simulink library "LDM_Controller"  (R2018b)
settings: Solver=VariableStepAuto  StartTime=0.0  StopTime=10.0  RelTol=1e-3
values from neighbouring files (symbols this model uses):
  K10_LDM_aOLCtrlerTableX : value not decoded    [LDM_DataDict.sldd]
  K10_LDM_torqOLCtrlerTableY : value not decoded    [LDM_DataDict.sldd]
  K_LDM_torqDecelClsCtrlerLowLim = -1000.0    [LDM_DataDict.sldd]
  K_LDM_torqDecelClsCtrlerUpLim = 1000.0    [LDM_DataDict.sldd]
  K_LDM_torqDecelCtrlerLowLim = 0.0    [LDM_DataDict.sldd]
  K_LDM_torqDecelCtrlerUpLim = 20000.0    [LDM_DataDict.sldd]
  K_LDM_torqOLCtrlerDecRate = 2.0    [LDM_DataDict.sldd]
  K_LDM_torqOLCtrlerIncRate = 2.0    [LDM_DataDict.sldd]
  K_LDM_torqOLCtrlerLowLim = 0.0    [LDM_DataDict.sldd]
  K_LDM_torqOLCtrlerResetLim = 10.0    [LDM_DataDict.sldd]
  K_LDM_torqOLCtrlerUpLim = 20000.0    [LDM_DataDict.sldd]
  LDM_VLD_EN_T : value not decoded    [LDM_DataDict.sldd]
  LDMCtrlMode_en_t : value not decoded    [LDM_DataDict.sldd]
undefined symbols (not defined in the file or in its folder): DiscIntNeverNeededParam
libraries: simulink x12
(part 2 of 2)

== stateflow chart LDM_Controller/Switch-Hybird Controller/LDM_Arbitrator ==
  state Decel_Control
    en:
    V_LDM_resetCtrler_bl = false;
    V_LDM_coHighSpdP = K_LDM_coDecelCtrlHighSpd_P;
    V_LDM_coHighSpdI = K_LDM_coDecelCtrlHighSpd_I;
    V_LDM_coLowSpdP = K_LDM_coDecelCtrlLowSpd_P;
    V_LDM_coLowSpdI = K_LDM_coDecelCtrlLowSpd_I;
    % PI parameters for DBR CST
    V_LDM_coCSTP = K_LDM_coDecelCtrlCST_P;
    V_LDM_coCSTI = K_LDM_coDecelCtrlCST_I;
    % PI parameters for EBR Self Brake
    V_LDM_coEbrSlfBrkP = K_LDM_coDecelCtrlEbrSB_P;
    V_LDM_coEbrSlfBrkI = K_LDM_coDecelCtrlEbrSB_I;
    state Standby
      % No brake request current VehAcc as the default value
      V_LDM_stBrkSrcMode_en = LDM_BRK_SRC_MODE_EN_T.BTA_PEDAL_BRAKE_NONE;
      V_LDM_aCtrlerSetpoint_f32 = single(0);
      V_LDM_coCtrlerPCoeff_f32 = single(0);
      V_LDM_coCtrlerICoeff_f32 = single(0);
      V_LDM_aCtrlErr_f32 = single(0);
      V_LDM_stBrkArbMode_en = LDMBrkArbMode_en_t.Standby;
      ex:
      V_LDM_resetCtrlerVal=single(V_LDM_PrvCtrlerOut);
    state EBR_control
      V_LDM_stBrkSrcMode_en = LDM_BRK_SRC_MODE_EN_T.BTA_EXTERNAL_BRAKE;
      V_LDM_aCtrlerSetpoint_f32 = V_EBR_aCHACCDecelReq;
      if V_LDM_stVehFwBw_en >= 0
      % moving forward or hold
      V_LDM_aVehAccDecLong = -V_VDS_aVehAccLong;
      else
      % moving backward
      V_LDM_aVehAccDecLong = V_VDS_aVehAccLong;
      end
      state EBR_Standby
        V_LDM_stBrkArbMode_en = LDMBrkArbMode_en_t.EBR_Standby;
        V_LDM_stCtrlMode_en = LDMCtrlMode_en_t.DecelCtrl;
        V_LDM_aCtrlerSetpoint_f32 = single(0);
        V_LDM_coCtrlerPCoeff_f32 = single(0);
        V_LDM_coCtrlerICoeff_f32 = single(0);
        V_LDM_aCtrlErr_f32 = single(0);
        V_LDM_resetCtrlerVal = single(0);
        V_LDM_resetCtrler_bl=~V_LDM_resetCtrler_bl;
      state EBR_DecelCtrl
        state DecelCtrl_CL_HighSpd
          en:
          V_LDM_stCtrlMode_en = LDMCtrlMode_en_t.DecelCtrl;
          V_LDM_coCtrlerPCoeff_f32 = V_LDM_coHighSpdP;
          V_LDM_coCtrlerICoeff_f32 = V_LDM_coHighSpdI;
          V_LDM_aCtrlErr_f32 = V_LDM_aCtrlerSetpoint_f32-V_LDM_aVehAccDecLong;
          V_LDM_resetCtrlerVal=V_LDM_PrvCtrlerOut-V_LDM_coCtrlerPCoeff_f32*V_LDM_aCtrlErr_f32;
          V_LDM_resetCtrler_bl=~V_LDM_resetCtrler_bl;
          du:
          V_LDM_aCtrlErr_f32 = V_LDM_aCtrlerSetpoint_f32-V_LDM_aVehAccDecLong;
        state DecelCtrl_CL_LowSpd
          en:
          V_LDM_stCtrlMode_en = LDMCtrlMode_en_t.DecelCtrl;
          V_LDM_coCtrlerPCoeff_f32 = V_LDM_coLowSpdP;
          V_LDM_coCtrlerICoeff_f32 = V_LDM_coLowSpdI;
          V_LDM_aCtrlErr_f32 = V_LDM_aCtrlerSetpoint_f32-V_LDM_aVehAccDecLong;
          V_LDM_resetCtrlerVal=V_LDM_PrvCtrlerOut-V_LDM_coCtrlerPCoeff_f32*V_LDM_aCtrlErr_f32;
          V_LDM_resetCtrler_bl=~V_LDM_resetCtrler_bl;
          du:
          V_LDM_aCtrlErr_f32 = V_LDM_aCtrlerSetpoint_f32-V_LDM_aVehAccDecLong;
        state DecelCtrl_OL
          en:
          V_LDM_stCtrlMode_en = LDMCtrlMode_en_t.OLCtrl; % open-loop control
          V_LDM_coCtrlerPCoeff_f32 = 0;
          V_LDM_coCtrlerICoeff_f32 = 0;
          V_LDM_resetCtrlerVal=V_LDM_PrvCtrlerOut;
          V_LDM_resetCtrler_bl=~V_LDM_resetCtrler_bl;
        (junction 414) -> Decel_Control.EBR_control.EBR_DecelCtrl.DecelCtrl_CL_HighSpd
        (junction 412) -> (junction 414) [order 2]
        Decel_Control.EBR_control.EBR_DecelCtrl.DecelCtrl_CL_HighSpd -> Decel_Control.EBR_control.EBR_DecelCtrl.DecelCtrl_CL_LowSpd : [abs(V_VDS_velVehSpd) <= K_LDM_coDecelCtrlHigh2LowLim]
        Decel_Control.EBR_control.EBR_DecelCtrl.DecelCtrl_CL_LowSpd -> Decel_Control.EBR_control.EBR_DecelCtrl.DecelCtrl_CL_HighSpd [order 2] : [abs(V_VDS_velVehSpd) > K_LDM_coDecelCtrlLow2HighLim]
        (junction 412) -> Decel_Control.EBR_control.EBR_DecelCtrl.DecelCtrl_CL_LowSpd [order 1] : [abs(V_VDS_velVehSpd) <= K_LDM_coDecelCtrlHigh2LowLim]
        (junction 411) -> (junction 412) [order 2]
        Decel_Control.EBR_control.EBR_DecelCtrl.DecelCtrl_OL -> Decel_Control.EBR_control.EBR_DecelCtrl.DecelCtrl_CL_LowSpd : [abs(V_VDS_velVehSpd) > K_LDM_coDecelCtrlOl2ClLim && ...
            | K_LDM_blClsLoopCtrlEnable_bl == true]
        Decel_Control.EBR_control.EBR_DecelCtrl.DecelCtrl_CL_LowSpd -> Decel_Control.EBR_control.EBR_DecelCtrl.DecelCtrl_OL [order 1] : [abs(V_VDS_velVehSpd) <= K_LDM_coDecelCtrlCl2OlLim]
        (junction 411) -> Decel_Control.EBR_control.EBR_DecelCtrl.DecelCtrl_OL [order 1] : [abs(V_VDS_velVehSpd) <= K_LDM_coDecelCtrlCl2OlLim || ...
            | K_LDM_blClsLoopCtrlEnable_bl == false]
        (default) -> (junction 411)
      state SelfBrake
        V_LDM_aCtrlErr_f32 = V_LDM_aCtrlerSetpoint_f32-V_LDM_aVehAccDecLong;
        state SelfBrake_follow
          en:
          V_LDM_stCtrlMode_en = LDMCtrlMode_en_t.DecelCtrl;
          V_LDM_coCtrlerPCoeff_f32 = V_LDM_coEbrSlfBrkP;
          V_LDM_coCtrlerICoeff_f32 = V_LDM_coEbrSlfBrkI;
          V_LDM_resetCtrlerVal=V_LDM_PrvCtrlerOut-V_LDM_coCtrlerPCoeff_f32*V_LDM_aCtrlErr_f32;
          V_LDM_resetCtrler_bl=~V_LDM_resetCtrler_bl;
        state StableJudge
          en:
          V_LDM_stCtrlMode_en = LDMCtrlMode_en_t.OLCtrl; % open-loop control
          V_LDM_coCtrlerPCoeff_f32 = 0;
          V_LDM_coCtrlerICoeff_f32 = 0;
          V_LDM_resetCtrlerVal=V_LDM_PrvCtrlerOut;
          V_LDM_resetCtrler_bl=~V_LDM_resetCtrler_bl;
        (junction 426) -> SelfBrake_follow
        (junction 424) -> (junction 426) [order 2]
        SelfBrake_follow -> StableJudge : [abs(V_VDS_velVehSpd) <= K_LDM_coDecelCtrlCl2OlLim]
        StableJudge -> SelfBrake_follow : [abs(V_VDS_velVehSpd) > K_LDM_coDecelCtrlOl2ClLim && ...
            | K_LDM_blClsLoopCtrlEnable_bl == true]
        (junction 424) -> StableJudge [order 1] : [abs(V_VDS_velVehSpd) <= K_LDM_coDecelCtrlCl2OlLim || ...
            | K_LDM_blClsLoopCtrlEnable_bl == false]
        (default) -> (junction 424)
      state HoldPressure
        en:
        V_LDM_stCtrlMode_en = LDMCtrlMode_en_t.OLCtrl;
        V_LDM_coCtrlerPCoeff_f32 = 0;
        V_LDM_coCtrlerICoeff_f32 = 0;
        V_LDM_resetCtrlerVal=V_LDM_PrvCtrlerOut;
        V_LDM_resetCtrler_bl=~V_LDM_resetCtrler_bl;
      (default) -> (junction 128)
      (junction 128) -> EBR_Standby [order 1] : [V_EBR_stCHACCRunbleSts_en == CHACCRunbleSts_en_t.ACC_standby]
      EBR_Standby -> EBR_control : [V_EBR_stCHACCRunbleSts_en ~= CHACCRunbleSts_en_t.ACC_standby]
      (junction 128) -> (junction 150) [order 2]
      (junction 225) -> EBR_Standby
      (junction 226) -> (junction 225) : {V_LDM_stBrkArbMode_en = LDMBrkArbMode_en_t.EBR_Error;}%error
      (junction 150) -> EBR_DecelCtrl [order 1] : [V_EBR_stCHACCRunbleSts_en == CHACCRunbleSts_en_t.ACC_CB]
          | {V_LDM_stBrkArbMode_en = LDMBrkArbMode_en_t.EBR_NormCtrl;}
      (junction 150) -> (junction 291) [order 2]
      EBR_DecelCtrl -> EBR_control : [V_EBR_stCHACCRunbleSts_en ~= CHACCRunbleSts_en_t.ACC_CB]
      (junction 291) -> SelfBrake [order 1] : [V_EBR_stCHACCRunbleSts_en == CHACCRunbleSts_en_t.ACC_SB]
          | {V_LDM_stBrkArbMode_en = LDMBrkArbMode_en_t.EBR_SelfBrake;}
      (junction 291) -> (junction 149) [order 2]
      SelfBrake -> EBR_control : [V_EBR_stCHACCRunbleSts_en ~= CHACCRunbleSts_en_t.ACC_SB]
      Decel_Control.EBR_control.HoldPressure -> EBR_control : [V_EBR_stCHACCRunbleSts_en ~= CHACCRunbleSts_en_t.ACC_HOLD]
      (junction 149) -> Decel_Control.EBR_control.HoldPressure [order 1] : [V_EBR_stCHACCRunbleSts_en == CHACCRunbleSts_en_t.ACC_HOLD]
      (junction 149) -> (junction 226) [order 2]
    state DBR_control
      V_LDM_stBrkSrcMode_en = LDM_BRK_SRC_MODE_EN_T.BTA_PEDAL_APPLIED;
      V_LDM_aCtrlerSetpoint_f32 = V_DBR_aDBRDecelReq;
      if V_LDM_stVehFwBw_en >= 0
      % moving forward or hold
      V_LDM_aVehAccDecLong = -V_VDS_aVehAccLong;
      else
      % moving backward
      V_LDM_aVehAccDecLong = V_VDS_aVehAccLong;
      end
      state initial
        V_LDM_stBrkArbMode_en = LDMBrkArbMode_en_t.DBR_Init;
      state DBR_DecelCtrl
        state DecelCtrl_CL_HighSpd
          en:
          V_LDM_stCtrlMode_en = LDMCtrlMode_en_t.DecelCtrl;
          V_LDM_coCtrlerPCoeff_f32 = V_LDM_coHighSpdP;
          V_LDM_coCtrlerICoeff_f32 = V_LDM_coHighSpdI;
          V_LDM_aCtrlErr_f32 = V_LDM_aCtrlerSetpoint_f32-V_LDM_aVehAccDecLong;
          V_LDM_resetCtrlerVal=V_LDM_PrvCtrlerOut-V_LDM_coCtrlerPCoeff_f32*V_LDM_aCtrlErr_f32;
          V_LDM_resetCtrler_bl=~V_LDM_resetCtrler_bl;
          du:
          V_LDM_aCtrlErr_f32 = V_LDM_aCtrlerSetpoint_f32-V_LDM_aVehAccDecLong;
        state DecelCtrl_CL_LowSpd
          en:
          V_LDM_stCtrlMode_en = LDMCtrlMode_en_t.DecelCtrl;
          V_LDM_coCtrlerPCoeff_f32 = V_LDM_coLowSpdP;
          V_LDM_coCtrlerICoeff_f32 = V_LDM_coLowSpdI;
          V_LDM_aCtrlErr_f32 = V_LDM_aCtrlerSetpoint_f32-V_LDM_aVehAccDecLong;
          V_LDM_resetCtrlerVal=V_LDM_PrvCtrlerOut-V_LDM_coCtrlerPCoeff_f32*V_LDM_aCtrlErr_f32;
          V_LDM_resetCtrler_bl=~V_LDM_resetCtrler_bl;
          du:
          V_LDM_aCtrlErr_f32 = V_LDM_aCtrlerSetpoint_f32-V_LDM_aVehAccDecLong;
        state DecelCtrl_OL
          en:
          V_LDM_stCtrlMode_en = LDMCtrlMode_en_t.OLCtrl; % open-loop control
          V_LDM_coCtrlerPCoeff_f32 = 0;
          V_LDM_coCtrlerICoeff_f32 = 0;
          V_LDM_resetCtrlerVal=V_LDM_PrvCtrlerOut;
          V_LDM_resetCtrler_bl=~V_LDM_resetCtrler_bl;
        (junction 389) -> Decel_Control.DBR_control.DBR_DecelCtrl.DecelCtrl_CL_HighSpd
        (junction 391) -> (junction 389) [order 2]
        Decel_Control.DBR_control.DBR_DecelCtrl.DecelCtrl_CL_HighSpd -> Decel_Control.DBR_control.DBR_DecelCtrl.DecelCtrl_CL_LowSpd : [abs(V_VDS_velVehSpd) <= K_LDM_coDecelCtrlHigh2LowLim]
        Decel_Control.DBR_control.DBR_DecelCtrl.DecelCtrl_CL_LowSpd -> Decel_Control.DBR_control.DBR_DecelCtrl.DecelCtrl_CL_HighSpd [order 2] : [abs(V_VDS_velVehSpd) > K_LDM_coDecelCtrlLow2HighLim]
        (junction 391) -> Decel_Control.DBR_control.DBR_DecelCtrl.DecelCtrl_CL_LowSpd [order 1] : [abs(V_VDS_velVehSpd) <= K_LDM_coDecelCtrlHigh2LowLim]
        (junction 393) -> (junction 391) [order 2]
        Decel_Control.DBR_control.DBR_DecelCtrl.DecelCtrl_OL -> Decel_Control.DBR_control.DBR_DecelCtrl.DecelCtrl_CL_LowSpd : [abs(V_VDS_velVehSpd) > K_LDM_coDecelCtrlOl2ClLim && ...
            | K_LDM_blClsLoopCtrlEnable_bl == true]
        Decel_Control.DBR_control.DBR_DecelCtrl.DecelCtrl_CL_LowSpd -> Decel_Control.DBR_control.DBR_DecelCtrl.DecelCtrl_OL [order 1] : [abs(V_VDS_velVehSpd) <= K_LDM_coDecelCtrlCl2OlLim]
        (junction 393) -> Decel_Control.DBR_control.DBR_DecelCtrl.DecelCtrl_OL [order 1] : [abs(V_VDS_velVehSpd) <= K_LDM_coDecelCtrlCl2OlLim || ...
            | K_LDM_blClsLoopCtrlEnable_bl == false]
        (default) -> (junction 393)
      state DBR_CST
        V_LDM_aCtrlErr_f32 = V_LDM_aCtrlerSetpoint_f32-V_LDM_aVehAccDecLong;
        state CST_follow
          en:
          V_LDM_stCtrlMode_en = LDMCtrlMode_en_t.DecelCtrl;
          V_LDM_coCtrlerPCoeff_f32 = V_LDM_coCSTP;
          V_LDM_coCtrlerICoeff_f32 = V_LDM_coCSTI;
          V_LDM_resetCtrlerVal=V_LDM_PrvCtrlerOut-V_LDM_coCtrlerPCoeff_f32*V_LDM_aCtrlErr_f32;
          V_LDM_resetCtrler_bl=~V_LDM_resetCtrler_bl;
        state CST_OL
          en:
          V_LDM_stCtrlMode_en = LDMCtrlMode_en_t.OLCtrl; % open-loop control
          V_LDM_coCtrlerPCoeff_f32 = 0;
          V_LDM_coCtrlerICoeff_f32 = 0;
          V_LDM_resetCtrlerVal=V_LDM_PrvCtrlerOut;
          V_LDM_resetCtrler_bl=~V_LDM_resetCtrler_bl;
        (junction 421) -> CST_follow
        (junction 419) -> (junction 421) [order 2]
        CST_follow -> CST_OL : [abs(V_VDS_velVehSpd) <= K_LDM_coDecelCtrlCl2OlLim]
        CST_OL -> CST_follow : [abs(V_VDS_velVehSpd) >= K_LDM_coDecelCtrlOl2ClLim && ...
            | K_LDM_blClsLoopCtrlEnable_bl == true]
        (junction 419) -> CST_OL [order 1] : [abs(V_VDS_velVehSpd) <= K_LDM_coDecelCtrlCl2OlLim || ...
            | K_LDM_blClsLoopCtrlEnable_bl == false]
        (default) -> (junction 419)
      state HoldPressure
        en:
        V_LDM_stBrkArbMode_en = LDMBrkArbMode_en_t.DBR_HldPres;
        V_LDM_stCtrlMode_en = LDMCtrlMode_en_t.OLCtrl;
        V_LDM_coCtrlerPCoeff_f32 = 0;
        V_LDM_coCtrlerICoeff_f32 = 0;
        V_LDM_resetCtrlerVal=V_LDM_PrvCtrlerOut;
        V_LDM_resetCtrler_bl=~V_LDM_resetCtrler_bl;
      (default) -> (junction 211)
      initial -> DBR_control : [V_DBR_stDBRRunbleSts_en ~= DBRCSTRunbleSts_en_t.initial]
      (junction 211) -> initial [order 1] : [V_DBR_stDBRRunbleSts_en == DBRCSTRunbleSts_en_t.initial]
      (junction 211) -> (junction 181) [order 2]
      (junction 181) -> DBR_DecelCtrl [order 1] : [V_DBR_stDBRRunbleSts_en == DBRCSTRunbleSts_en_t.CST_emergency_control]
          | {V_LDM_stBrkArbMode_en = LDMBrkArbMode_en_t.DBR_EmergCtrl;}
      (junction 181) -> (junction 180) [order 2]
      DBR_DecelCtrl -> DBR_control : [V_DBR_stDBRRunbleSts_en ~= DBRCSTRunbleSts_en_t.dynamic_control &&...
          | V_DBR_stDBRRunbleSts_en ~= DBRCSTRunbleSts_en_t.CST_standby_dynamic_control &&...
          | V_DBR_stDBRRunbleSts_en ~= DBRCSTRunbleSts_en_t.CST_emergency_control]
      (junction 180) -> DBR_DecelCtrl [order 1] : [V_DBR_stDBRRunbleSts_en == DBRCSTRunbleSts_en_t.dynamic_control ||...
          | V_DBR_stDBRRunbleSts_en == DBRCSTRunbleSts_en_t.CST_standby_dynamic_control]
          | {V_LDM_stBrkArbMode_en = LDMBrkArbMode_en_t.DBR_NormCtrl;}
      (junction 180) -> (junction 182) [order 2]
      (junction 262) -> DBR_DecelCtrl
      (junction 260) -> (junction 262) : {V_LDM_stBrkArbMode_en = LDMBrkArbMode_en_t.DBR_Error;}%error
      DBR_CST -> DBR_control : [V_DBR_stDBRRunbleSts_en ~= DBRCSTRunbleSts_en_t.CST_active]
      (junction 182) -> DBR_CST [order 1] : [V_DBR_stDBRRunbleSts_en == DBRCSTRunbleSts_en_t.CST_active]
          | {V_LDM_stBrkArbMode_en = LDMBrkArbMode_en_t.DBR_CST;}
      (junction 182) -> (junction 273) [order 2]
      Decel_Control.DBR_control.HoldPressure -> DBR_control : [V_DBR_stDBRRunbleSts_en ~= DBRCSTRunbleSts_en_t.CST_off && ...
          | V_DBR_stDBRRunbleSts_en ~= DBRCSTRunbleSts_en_t.CST_standby_standstill_control &&...
          | V_DBR_stDBRRunbleSts_en ~= DBRCSTRunbleSts_en_t.standstill_control]
      (junction 273) -> Decel_Control.DBR_control.HoldPressure [order 1] : [V_DBR_stDBRRunbleSts_en == DBRCSTRunbleSts_en_t.CST_off ||...
          | V_DBR_stDBRRunbleSts_en == DBRCSTRunbleSts_en_t.CST_standby_standstill_control ||...
          | V_DBR_stDBRRunbleSts_en == DBRCSTRunbleSts_en_t.standstill_control]
      (junction 273) -> (junction 260) [order 2]
    DBR_control -> Standby [order 1] : [V_DBR_EBR_stBrkArbMode_en==BrkArbMode_en_t.brake_no_request]
        | {V_LDM_resetCtrler_bl=~V_LDM_resetCtrler_bl; V_LDM_resetCtrlerVal=single(0);}
    EBR_control -> Standby [order 1] : [V_DBR_EBR_stBrkArbMode_en==BrkArbMode_en_t.brake_no_request]
        | {V_LDM_resetCtrler_bl=~V_LDM_resetCtrler_bl; V_LDM_resetCtrlerVal=single(0);}
    Standby -> DBR_control [order 1] : [V_DBR_EBR_stBrkArbMode_en==BrkArbMode_en_t.DBR_arbitration]
    Standby -> EBR_control [order 2] : [V_DBR_EBR_stBrkArbMode_en==BrkArbMode_en_t.ACC_arbitration && ...
        | V_EBR_stCHACCRunbleSts_en ~= CHACCRunbleSts_en_t.ACC_off]
    (junction 71) -> Standby [order 3]
    (junction 71) -> EBR_control [order 2] : [V_DBR_EBR_stBrkArbMode_en==BrkArbMode_en_t.ACC_arbitration]
    (junction 71) -> DBR_control [order 1] : [V_DBR_EBR_stBrkArbMode_en==BrkArbMode_en_t.DBR_arbitration]
    (default) -> (junction 71)
    DBR_control -> EBR_control [order 2] : [V_DBR_EBR_stBrkArbMode_en==BrkArbMode_en_t.ACC_arbitration]
    EBR_control -> DBR_control [order 2] : [V_DBR_EBR_stBrkArbMode_en==BrkArbMode_en_t.DBR_arbitration]
  (default) -> Decel_Control
  data: V_LDM_stCtrlMode_en output; V_LDM_aCtrlErr_f32 output; V_DBR_EBR_stBrkArbMode_en input Enum: BrkArbMode_en_t; V_LDM_stVehFwBw_en input Enum: LDMVehFwBw_en_t; V_DBR_aDBRDecelReq input single; V_EBR_aCHACCDecelReq input single; V_DBR_stDBRRunbleSts_en input Enum: DBRCSTRunbleSts_en_t; V_EBR_stCHACCRunbleSts_en input Enum: CHACCRunbleSts_en_t; V_VDS_aVehAccLong input single; V_VDS_velVehSpd input single; V_LDM_coCtrlerPCoeff_f32 output single; V_LDM_coCtrlerICoeff_f32 output single; V_LDM_resetCtrler_bl output boolean; V_LDM_resetCtrlerVal output single; V_LDM_PrvCtrlerOut input single; V_LDM_aCtrlerSetpoint_f32 output single; V_LDM_coHighSpdI local single; V_LDM_coHighSpdP local single; V_LDM_coCSTI local single; V_LDM_aVehAccDecLong local single; V_LDM_coCSTP local; V_LDM_stBrkArbMode_en output; K_LDM_coDecelCtrlCST_I parameter; K_LDM_coDecelCtrlCST_P parameter; V_LDM_coEbrSlfBrkP local; V_LDM_coEbrSlfBrkI local; K_LDM_coDecelCtrlEbrSB_I parameter; K_LDM_coDecelCtrlEbrSB_P parameter; V_LDM_coLowSpdI local; V_LDM_coLowSpdP local; K_LDM_coDecelCtrlHighSpd_I parameter; K_LDM_coDecelCtrlLowSpd_I parameter; K_LDM_coDecelCtrlHighSpd_P parameter; K_LDM_coDecelCtrlLowSpd_P parameter; K_LDM_coDecelCtrlCl2OlLim parameter; K_LDM_coDecelCtrlHigh2LowLim parameter; K_LDM_coDecelCtrlLow2HighLim parameter; K_LDM_coDecelCtrlOl2ClLim parameter; K_LDM_blClsLoopCtrlEnable_bl parameter; V_LDM_stBrkSrcMode_en output

== stateflow chart LDM_Controller/Switch-Hybird Controller/Decel open-loop controler1/reset ==
  state CalDiff
    en:
    if PrevCtrlOutput <= 0.1 || K_LDM_blClsLoopCtrlEnable_bl == false
    %previous control output equals zero, or closed loop control is unabled
    eta = 1;
    else
    eta = PrevCtrlOutput / max(1, LookupTableValue);
    end
  state Hold
  (default) -> CalDiff
  CalDiff -> Hold : [~enable]
  Hold -> CalDiff : [enable]
  data: enable input boolean; LookupTableValue input single; PrevCtrlOutput input single; eta output single; K_LDM_blClsLoopCtrlEnable_bl parameter

== stateflow chart LDM_Controller/Parallel-Hybird Controller/Decel open-loop controler1/reset ==
  state CalDiff
    en:
    if PrevCtrlOutput <= 0.1 || K_LDM_blClsLoopCtrlEnable_bl == false
    %previous control output equals zero, or closed loop control is unabled
    eta = 1;
    else
    eta = PrevCtrlOutput / max(1, LookupTableValue);
    end
  state Hold
  (default) -> CalDiff
  CalDiff -> Hold : [~enable]
  Hold -> CalDiff : [enable]
  data: enable input boolean; LookupTableValue input single; PrevCtrlOutput input single; eta output single; K_LDM_blClsLoopCtrlEnable_bl parameter

== stateflow chart LDM_Controller/Parallel-Hybird Controller/LDM_Arbitrator ==
  state Decel_Control
    en:
    V_LDM_resetCtrler_bl = false;
    V_LDM_coHighSpdP = K_LDM_coDecelParalCtrlHighSpd_P;
    V_LDM_coHighSpdI = K_LDM_coDecelParalCtrlHighSpd_I;
    V_LDM_coLowSpdP = K_LDM_coDecelParalCtrlLowSpd_P;
    V_LDM_coLowSpdI = K_LDM_coDecelParalCtrlLowSpd_I;
    % PI parameters for DBR CST
    V_LDM_coCSTP = K_LDM_coDecelParalCtrlCST_P;
    V_LDM_coCSTI = K_LDM_coDecelParalCtrlCST_I;
    % PI parameters for EBR Self Brake
    V_LDM_coEbrSlfBrkP = K_LDM_coDecelParalCtrlEbrSB_P;
    V_LDM_coEbrSlfBrkI = K_LDM_coDecelParalCtrlEbrSB_I;
    du:
    % whether enable the closed loop controller
    if K_LDM_blClsLoopCtrlEnable_bl == false
    V_LDM_stClsLoopEnable = false;
    else
    if V_LDM_stVehFwBw_en == LDMVehFwBw_en_t.Forward ||...
    V_LDM_stVehFwBw_en == LDMVehFwBw_en_t.Backward
    V_LDM_stClsLoopEnable = true;
    else
    V_LDM_stClsLoopEnable = false;
    end
    end
    % moving forward
    if V_LDM_stVehFwBw_en == LDMVehFwBw_en_t.Forward
    V_LDM_aVehAccDecLong = -V_VDS_aVehAccLong;
    % moving backward
    elseif V_LDM_stVehFwBw_en == LDMVehFwBw_en_t.Backward
    V_LDM_aVehAccDecLong = V_VDS_aVehAccLong;
    else
    V_LDM_aVehAccDecLong = V_VDS_aVehAccLong;
    end
    V_LDM_aVehAccErr = V_LDM_aCtrlerSetpoint_f32-V_LDM_aVehAccDecLong;
    state Standby
      % No brake request current VehAcc as the default value
      V_LDM_stBrkSrcMode_en = LDM_BRK_SRC_MODE_EN_T.BTA_PEDAL_BRAKE_NONE;
      V_LDM_aCtrlerSetpoint_f32 = single(0);
      V_LDM_coCtrlerPCoeff_f32 = single(0);
      V_LDM_coCtrlerICoeff_f32 = single(0);
      V_LDM_aCtrlErr_f32 = single(0);
      V_LDM_stBrkArbMode_en = LDMBrkArbMode_en_t.Standby;
      en:
      V_LDM_resetCtrlerVal = single(0);
      V_LDM_resetCtrler_bl=~V_LDM_resetCtrler_bl;
      ex:
      V_LDM_resetCtrlerVal=single(V_LDM_PrvClsLoopCtrlerOut);
    state DBR_control
      V_LDM_stBrkSrcMode_en = LDM_BRK_SRC_MODE_EN_T.BTA_PEDAL_APPLIED;
      V_LDM_aCtrlerSetpoint_f32 = V_DBR_aDBRDecelReq;
      state initial
        V_LDM_stBrkArbMode_en = LDMBrkArbMode_en_t.DBR_Init;
        V_LDM_stCtrlMode_en = LDMCtrlMode_en_t.OLCtrl;
      state DBR_DecelCtrl
        state DecelCtrl_CL_HighSpd
          en,du:
          V_LDM_aCtrlErr_f32 = V_LDM_aVehAccErr;
          en:
          V_LDM_stCtrlMode_en = LDMCtrlMode_en_t.DecelCtrl;
          V_LDM_coCtrlerPCoeff_f32 = V_LDM_coHighSpdP;
          V_LDM_coCtrlerICoeff_f32 = V_LDM_coHighSpdI;
          V_LDM_resetCtrlerVal=V_LDM_PrvClsLoopCtrlerOut-V_LDM_coCtrlerPCoeff_f32*V_LDM_aCtrlErr_f32;
          V_LDM_resetCtrler_bl=~V_LDM_resetCtrler_bl;
        state DecelCtrl_CL_LowSpd
          en,du:
          V_LDM_aCtrlErr_f32 = V_LDM_aVehAccErr;
          en:
          V_LDM_stCtrlMode_en = LDMCtrlMode_en_t.DecelCtrl;
          V_LDM_coCtrlerPCoeff_f32 = V_LDM_coLowSpdP;
          V_LDM_coCtrlerICoeff_f32 = V_LDM_coLowSpdI;
          V_LDM_resetCtrlerVal=V_LDM_PrvClsLoopCtrlerOut-V_LDM_coCtrlerPCoeff_f32*V_LDM_aCtrlErr_f32;
          V_LDM_resetCtrler_bl=~V_LDM_resetCtrler_bl;
        state DecelCtrl_OL
          en:
          V_LDM_coCtrlerPCoeff_f32 = 0;
          V_LDM_coCtrlerICoeff_f32 = V_LDM_coLowSpdI / V_LDM_coLowSpdP;
          V_LDM_resetCtrlerVal=V_LDM_PrvClsLoopCtrlerOut;
          V_LDM_resetCtrler_bl=~V_LDM_resetCtrler_bl;
          du:
          V_LDM_aCtrlErr_f32 = - V_LDM_PrvClsLoopCtrlerOut; % let cls ctrl go to zero smoothly
          if abs(V_LDM_PrvClsLoopCtrlerOut) <= 0.1
          V_LDM_stCtrlMode_en = LDMCtrlMode_en_t.OLCtrl; % open-loop control
          V_LDM_coCtrlerICoeff_f32 = 0;
          V_LDM_resetCtrlerVal=0;
          V_LDM_resetCtrler_bl=~V_LDM_resetCtrler_bl;
          end
        (junction 389) -> Decel_Control.DBR_control.DBR_DecelCtrl.DecelCtrl_CL_HighSpd
        (junction 391) -> (junction 389) [order 2]
        Decel_Control.DBR_control.DBR_DecelCtrl.DecelCtrl_CL_HighSpd -> Decel_Control.DBR_control.DBR_DecelCtrl.DecelCtrl_CL_LowSpd : [abs(V_VDS_velVehSpd) <= K_LDM_coDecelCtrlHigh2LowLim]
        Decel_Control.DBR_control.DBR_DecelCtrl.DecelCtrl_CL_LowSpd -> Decel_Control.DBR_control.DBR_DecelCtrl.DecelCtrl_CL_HighSpd [order 2] : [abs(V_VDS_velVehSpd) > K_LDM_coDecelCtrlLow2HighLim]
        (junction 391) -> Decel_Control.DBR_control.DBR_DecelCtrl.DecelCtrl_CL_LowSpd [order 1] : [abs(V_VDS_velVehSpd) <= K_LDM_coDecelCtrlHigh2LowLim]
        (junction 393) -> (junction 391) [order 2]
        Decel_Control.DBR_control.DBR_DecelCtrl.DecelCtrl_OL -> Decel_Control.DBR_control.DBR_DecelCtrl.DecelCtrl_CL_LowSpd : [abs(V_VDS_velVehSpd) > K_LDM_coDecelCtrlOl2ClLim && ...
            | V_LDM_stClsLoopEnable == true]
        Decel_Control.DBR_control.DBR_DecelCtrl.DecelCtrl_CL_LowSpd -> Decel_Control.DBR_control.DBR_DecelCtrl.DecelCtrl_OL [order 1] : [abs(V_VDS_velVehSpd) <= K_LDM_coDecelCtrlCl2OlLim]
        (junction 393) -> Decel_Control.DBR_control.DBR_DecelCtrl.DecelCtrl_OL [order 1] : [abs(V_VDS_velVehSpd) <= K_LDM_coDecelCtrlCl2OlLim || ...
            | V_LDM_stClsLoopEnable == false]
        (default) -> (junction 393)
      state DBR_CST
        state CST_follow
          en,du:
          V_LDM_aCtrlErr_f32 = V_LDM_aVehAccErr;
          en:
          V_LDM_stCtrlMode_en = LDMCtrlMode_en_t.DecelCtrl;
          V_LDM_coCtrlerPCoeff_f32 = V_LDM_coCSTP;
          V_LDM_coCtrlerICoeff_f32 = V_LDM_coCSTI;
          V_LDM_resetCtrlerVal=V_LDM_PrvClsLoopCtrlerOut-V_LDM_coCtrlerPCoeff_f32*V_LDM_aCtrlErr_f32;
          V_LDM_resetCtrler_bl=~V_LDM_resetCtrler_bl;
        state CST_OL
          en:
          V_LDM_resetCtrlerVal=V_LDM_PrvClsLoopCtrlerOut;
          V_LDM_resetCtrler_bl=~V_LDM_resetCtrler_bl;
          V_LDM_coCtrlerPCoeff_f32 = 0;
          V_LDM_coCtrlerICoeff_f32 = V_LDM_coCSTI / V_LDM_coCSTP;
          du:
          V_LDM_aCtrlErr_f32 = - V_LDM_PrvClsLoopCtrlerOut; % let cls ctrl go to zero smoothly
          if abs(V_LDM_PrvClsLoopCtrlerOut) <= 0.1
          V_LDM_stCtrlMode_en = LDMCtrlMode_en_t.OLCtrl; % open-loop control
          V_LDM_coCtrlerICoeff_f32 = 0;
          V_LDM_resetCtrlerVal=0;
          V_LDM_resetCtrler_bl=~V_LDM_resetCtrler_bl;
          end
        (junction 421) -> CST_follow
        (junction 419) -> (junction 421) [order 2]
        CST_follow -> CST_OL : [abs(V_VDS_velVehSpd) <= K_LDM_coDecelCtrlCl2OlLim]
        CST_OL -> CST_follow : [abs(V_VDS_velVehSpd) >= K_LDM_coDecelCtrlOl2ClLim && ...
            | V_LDM_stClsLoopEnable == true]
        (junction 419) -> CST_OL [order 1] : [abs(V_VDS_velVehSpd) <= K_LDM_coDecelCtrlCl2OlLim || ...
            | V_LDM_stClsLoopEnable == false]
        (default) -> (junction 419)
      state HoldPressure
        en:
        V_LDM_stBrkArbMode_en = LDMBrkArbMode_en_t.DBR_HldPres;
        V_LDM_stCtrlMode_en = LDMCtrlMode_en_t.OLCtrl;
        V_LDM_coCtrlerPCoeff_f32 = 0;
        V_LDM_coCtrlerICoeff_f32 = 0;
        V_LDM_resetCtrlerVal=0;
        V_LDM_resetCtrler_bl=~V_LDM_resetCtrler_bl;
      (default) -> (junction 211)
      initial -> DBR_control : [V_DBR_stDBRRunbleSts_en ~= DBRCSTRunbleSts_en_t.initial]
      (junction 211) -> initial [order 1] : [V_DBR_stDBRRunbleSts_en == DBRCSTRunbleSts_en_t.initial]
      (junction 211) -> (junction 181) [order 2]
      (junction 181) -> DBR_DecelCtrl [order 1] : [V_DBR_stDBRRunbleSts_en == DBRCSTRunbleSts_en_t.CST_emergency_control]
          | {V_LDM_stBrkArbMode_en = LDMBrkArbMode_en_t.DBR_EmergCtrl;}
      (junction 181) -> (junction 180) [order 2]
      DBR_DecelCtrl -> DBR_control : [V_DBR_stDBRRunbleSts_en ~= DBRCSTRunbleSts_en_t.dynamic_control &&...
          | V_DBR_stDBRRunbleSts_en ~= DBRCSTRunbleSts_en_t.CST_standby_dynamic_control &&...
          | V_DBR_stDBRRunbleSts_en ~= DBRCSTRunbleSts_en_t.CST_emergency_control]
      (junction 180) -> DBR_DecelCtrl [order 1] : [V_DBR_stDBRRunbleSts_en == DBRCSTRunbleSts_en_t.dynamic_control ||...
          | V_DBR_stDBRRunbleSts_en == DBRCSTRunbleSts_en_t.CST_standby_dynamic_control]
          | {V_LDM_stBrkArbMode_en = LDMBrkArbMode_en_t.DBR_NormCtrl;}
      (junction 180) -> (junction 182) [order 2]
      (junction 262) -> DBR_DecelCtrl
      (junction 260) -> (junction 262) : {V_LDM_stBrkArbMode_en = LDMBrkArbMode_en_t.DBR_Error;}%error
      DBR_CST -> DBR_control : [V_DBR_stDBRRunbleSts_en ~= DBRCSTRunbleSts_en_t.CST_active]
      (junction 182) -> DBR_CST [order 1] : [V_DBR_stDBRRunbleSts_en == DBRCSTRunbleSts_en_t.CST_active]
          | {V_LDM_stBrkArbMode_en = LDMBrkArbMode_en_t.DBR_CST;}
      (junction 182) -> (junction 273) [order 2]
      Decel_Control.DBR_control.HoldPressure -> DBR_control : [V_DBR_stDBRRunbleSts_en ~= DBRCSTRunbleSts_en_t.CST_off && ...
          | V_DBR_stDBRRunbleSts_en ~= DBRCSTRunbleSts_en_t.CST_standby_standstill_control &&...
          | V_DBR_stDBRRunbleSts_en ~= DBRCSTRunbleSts_en_t.standstill_control]
      (junction 273) -> Decel_Control.DBR_control.HoldPressure [order 1] : [V_DBR_stDBRRunbleSts_en == DBRCSTRunbleSts_en_t.CST_off ||...
          | V_DBR_stDBRRunbleSts_en == DBRCSTRunbleSts_en_t.CST_standby_standstill_control ||...
          | V_DBR_stDBRRunbleSts_en == DBRCSTRunbleSts_en_t.standstill_control]
      (junction 273) -> (junction 260) [order 2]
    state EBR_control
      V_LDM_stBrkSrcMode_en = LDM_BRK_SRC_MODE_EN_T.BTA_EXTERNAL_BRAKE;
      V_LDM_aCtrlerSetpoint_f32 = V_EBR_aCHACCDecelReq;
      state EBR_Standby
        V_LDM_stBrkArbMode_en = LDMBrkArbMode_en_t.EBR_Standby;
        V_LDM_stCtrlMode_en = LDMCtrlMode_en_t.OLCtrl;
        V_LDM_aCtrlerSetpoint_f32 = single(0);
        V_LDM_coCtrlerPCoeff_f32 = single(0);
        V_LDM_coCtrlerICoeff_f32 = single(0);
        V_LDM_aCtrlErr_f32 = single(0);
        V_LDM_resetCtrlerVal = single(0);
        V_LDM_resetCtrler_bl=~V_LDM_resetCtrler_bl;
      state EBR_DecelCtrl
        state DecelCtrl_CL_HighSpd
          V_LDM_aCtrlErr_f32 = V_LDM_aVehAccErr;
          en:
          V_LDM_stCtrlMode_en = LDMCtrlMode_en_t.DecelCtrl;
          V_LDM_coCtrlerPCoeff_f32 = V_LDM_coHighSpdP;
          V_LDM_coCtrlerICoeff_f32 = V_LDM_coHighSpdI;
          V_LDM_resetCtrlerVal=V_LDM_PrvClsLoopCtrlerOut-V_LDM_coCtrlerPCoeff_f32*V_LDM_aCtrlErr_f32;
          V_LDM_resetCtrler_bl=~V_LDM_resetCtrler_bl;
        state DecelCtrl_CL_LowSpd
          V_LDM_aCtrlErr_f32 = V_LDM_aVehAccErr;
          en:
          V_LDM_stCtrlMode_en = LDMCtrlMode_en_t.DecelCtrl;
          V_LDM_coCtrlerPCoeff_f32 = V_LDM_coLowSpdP;
          V_LDM_coCtrlerICoeff_f32 = V_LDM_coLowSpdI;
          V_LDM_resetCtrlerVal=V_LDM_PrvClsLoopCtrlerOut-V_LDM_coCtrlerPCoeff_f32*V_LDM_aCtrlErr_f32;
          V_LDM_resetCtrler_bl=~V_LDM_resetCtrler_bl;
        state DecelCtrl_OL
          en:
          V_LDM_resetCtrlerVal=V_LDM_PrvClsLoopCtrlerOut;
          V_LDM_resetCtrler_bl=~V_LDM_resetCtrler_bl;
          V_LDM_coCtrlerPCoeff_f32 = 0;
          V_LDM_coCtrlerICoeff_f32 = V_LDM_coLowSpdI / V_LDM_coLowSpdP;
          du:
          V_LDM_aCtrlErr_f32 = - V_LDM_PrvClsLoopCtrlerOut; % let cls ctrl go to zero smoothly
          if abs(V_LDM_PrvClsLoopCtrlerOut) <= 0.1
          V_LDM_stCtrlMode_en = LDMCtrlMode_en_t.OLCtrl; % open-loop control
          V_LDM_coCtrlerICoeff_f32 = 0;
          V_LDM_resetCtrlerVal=0;
          V_LDM_resetCtrler_bl=~V_LDM_resetCtrler_bl;
          end
        (junction 414) -> Decel_Control.EBR_control.EBR_DecelCtrl.DecelCtrl_CL_HighSpd
        (junction 412) -> (junction 414) [order 2]
        Decel_Control.EBR_control.EBR_DecelCtrl.DecelCtrl_CL_HighSpd -> Decel_Control.EBR_control.EBR_DecelCtrl.DecelCtrl_CL_LowSpd : [abs(V_VDS_velVehSpd) <= K_LDM_coDecelCtrlHigh2LowLim]
        Decel_Control.EBR_control.EBR_DecelCtrl.DecelCtrl_CL_LowSpd -> Decel_Control.EBR_control.EBR_DecelCtrl.DecelCtrl_CL_HighSpd [order 2] : [abs(V_VDS_velVehSpd) > K_LDM_coDecelCtrlLow2HighLim]
        (junction 412) -> Decel_Control.EBR_control.EBR_DecelCtrl.DecelCtrl_CL_LowSpd [order 1] : [abs(V_VDS_velVehSpd) <= K_LDM_coDecelCtrlHigh2LowLim]
        (junction 411) -> (junction 412) [order 2]
        Decel_Control.EBR_control.EBR_DecelCtrl.DecelCtrl_OL -> Decel_Control.EBR_control.EBR_DecelCtrl.DecelCtrl_CL_LowSpd : [abs(V_VDS_velVehSpd) > K_LDM_coDecelCtrlOl2ClLim && ...
            | K_LDM_blClsLoopCtrlEnable_bl == true]
        Decel_Control.EBR_control.EBR_DecelCtrl.DecelCtrl_CL_LowSpd -> Decel_Control.EBR_control.EBR_DecelCtrl.DecelCtrl_OL [order 1] : [abs(V_VDS_velVehSpd) <= K_LDM_coDecelCtrlCl2OlLim]
        (junction 411) -> Decel_Control.EBR_control.EBR_DecelCtrl.DecelCtrl_OL [order 1] : [abs(V_VDS_velVehSpd) <= K_LDM_coDecelCtrlCl2OlLim || ...
            | K_LDM_blClsLoopCtrlEnable_bl == false]
        (default) -> (junction 411)
      state SelfBrake
        state SelfBrake_follow
          V_LDM_aCtrlErr_f32 = V_LDM_aVehAccErr;
          en:
          V_LDM_stCtrlMode_en = LDMCtrlMode_en_t.DecelCtrl;
          V_LDM_coCtrlerPCoeff_f32 = V_LDM_coEbrSlfBrkP;
          V_LDM_coCtrlerICoeff_f32 = V_LDM_coEbrSlfBrkI;
          V_LDM_resetCtrlerVal=V_LDM_PrvClsLoopCtrlerOut-V_LDM_coCtrlerPCoeff_f32*V_LDM_aCtrlErr_f32;
          V_LDM_resetCtrler_bl=~V_LDM_resetCtrler_bl;
        state SelfBrake_OL
          en:
          V_LDM_resetCtrlerVal=V_LDM_PrvClsLoopCtrlerOut;
          V_LDM_resetCtrler_bl=~V_LDM_resetCtrler_bl;
          V_LDM_coCtrlerPCoeff_f32 = 0;
          V_LDM_coCtrlerICoeff_f32 = V_LDM_coEbrSlfBrkI / V_LDM_coEbrSlfBrkP;
          du:
          V_LDM_aCtrlErr_f32 = - V_LDM_PrvClsLoopCtrlerOut; % let cls ctrl go to zero smoothly
          if abs(V_LDM_PrvClsLoopCtrlerOut) <= 0.1
          V_LDM_stCtrlMode_en = LDMCtrlMode_en_t.OLCtrl; % open-loop control
          V_LDM_coCtrlerICoeff_f32 = 0;
          V_LDM_resetCtrlerVal=0;
          V_LDM_resetCtrler_bl=~V_LDM_resetCtrler_bl;
          end
        (junction 426) -> SelfBrake_follow
        (junction 424) -> (junction 426) [order 2]
        SelfBrake_follow -> SelfBrake_OL : [abs(V_VDS_velVehSpd) <= K_LDM_coDecelCtrlCl2OlLim]
        SelfBrake_OL -> SelfBrake_follow : [abs(V_VDS_velVehSpd) > K_LDM_coDecelCtrlOl2ClLim && ...
            | K_LDM_blClsLoopCtrlEnable_bl == true]
        (junction 424) -> SelfBrake_OL [order 1] : [abs(V_VDS_velVehSpd) <= K_LDM_coDecelCtrlCl2OlLim || ...
            | K_LDM_blClsLoopCtrlEnable_bl == false]
        (default) -> (junction 424)
      state HoldPressure
        en:
        V_LDM_stCtrlMode_en = LDMCtrlMode_en_t.OLCtrl;
        V_LDM_coCtrlerPCoeff_f32 = 0;
        V_LDM_coCtrlerICoeff_f32 = 0;
        V_LDM_resetCtrlerVal=0;
        V_LDM_resetCtrler_bl=~V_LDM_resetCtrler_bl;
      (default) -> (junction 128)
      (junction 128) -> EBR_Standby [order 1] : [V_EBR_stCHACCRunbleSts_en == CHACCRunbleSts_en_t.ACC_standby]
      EBR_Standby -> EBR_control : [V_EBR_stCHACCRunbleSts_en ~= CHACCRunbleSts_en_t.ACC_standby]
      (junction 128) -> (junction 150) [order 2]
      (junction 225) -> EBR_Standby
      (junction 226) -> (junction 225) : {V_LDM_stBrkArbMode_en = LDMBrkArbMode_en_t.EBR_Error;}%error
      (junction 150) -> EBR_DecelCtrl [order 1] : [V_EBR_stCHACCRunbleSts_en == CHACCRunbleSts_en_t.ACC_CB]
          | {V_LDM_stBrkArbMode_en = LDMBrkArbMode_en_t.EBR_NormCtrl;}
      (junction 150) -> (junction 291) [order 2]
      EBR_DecelCtrl -> EBR_control : [V_EBR_stCHACCRunbleSts_en ~= CHACCRunbleSts_en_t.ACC_CB]
      (junction 291) -> SelfBrake [order 1] : [V_EBR_stCHACCRunbleSts_en == CHACCRunbleSts_en_t.ACC_SB]
          | {V_LDM_stBrkArbMode_en = LDMBrkArbMode_en_t.EBR_SelfBrake;}
      (junction 291) -> (junction 149) [order 2]
      SelfBrake -> EBR_control : [V_EBR_stCHACCRunbleSts_en ~= CHACCRunbleSts_en_t.ACC_SB]
      Decel_Control.EBR_control.HoldPressure -> EBR_control : [V_EBR_stCHACCRunbleSts_en ~= CHACCRunbleSts_en_t.ACC_HOLD]
      (junction 149) -> Decel_Control.EBR_control.HoldPressure [order 1] : [V_EBR_stCHACCRunbleSts_en == CHACCRunbleSts_en_t.ACC_HOLD]
      (junction 149) -> (junction 226) [order 2]
    DBR_control -> Standby [order 1] : [V_DBR_EBR_stBrkArbMode_en==BrkArbMode_en_t.brake_no_request]
        | {V_LDM_resetCtrler_bl=~V_LDM_resetCtrler_bl; V_LDM_resetCtrlerVal=single(0);}
    EBR_control -> Standby [order 1] : [V_DBR_EBR_stBrkArbMode_en==BrkArbMode_en_t.brake_no_request]
        | {V_LDM_resetCtrler_bl=~V_LDM_resetCtrler_bl; V_LDM_resetCtrlerVal=single(0);}
    Standby -> DBR_control [order 1] : [V_DBR_EBR_stBrkArbMode_en==BrkArbMode_en_t.DBR_arbitration]
    Standby -> EBR_control [order 2] : [V_DBR_EBR_stBrkArbMode_en==BrkArbMode_en_t.ACC_arbitration && ...
        | V_EBR_stCHACCRunbleSts_en ~= CHACCRunbleSts_en_t.ACC_off]
    (junction 71) -> Standby [order 3]
    (junction 71) -> EBR_control [order 2] : [V_DBR_EBR_stBrkArbMode_en==BrkArbMode_en_t.ACC_arbitration]
    (junction 71) -> DBR_control [order 1] : [V_DBR_EBR_stBrkArbMode_en==BrkArbMode_en_t.DBR_arbitration]
    (default) -> (junction 71)
    DBR_control -> EBR_control [order 2] : [V_DBR_EBR_stBrkArbMode_en==BrkArbMode_en_t.ACC_arbitration]
    EBR_control -> DBR_control [order 2] : [V_DBR_EBR_stBrkArbMode_en==BrkArbMode_en_t.DBR_arbitration]
  (default) -> Decel_Control
  data: V_LDM_stCtrlMode_en output; V_LDM_aCtrlErr_f32 output; V_DBR_EBR_stBrkArbMode_en input Enum: BrkArbMode_en_t; V_LDM_stVehFwBw_en input Enum: LDMVehFwBw_en_t; V_DBR_aDBRDecelReq input single; V_EBR_aCHACCDecelReq input single; V_DBR_stDBRRunbleSts_en input Enum: DBRCSTRunbleSts_en_t; V_EBR_stCHACCRunbleSts_en input Enum: CHACCRunbleSts_en_t; V_VDS_aVehAccLong input single; V_VDS_velVehSpd input single; V_LDM_coCtrlerPCoeff_f32 output single; V_LDM_coCtrlerICoeff_f32 output single; V_LDM_resetCtrler_bl output boolean; V_LDM_resetCtrlerVal output single; V_LDM_PrvClsLoopCtrlerOut input single; V_LDM_aCtrlerSetpoint_f32 output single; V_LDM_coHighSpdI local single; V_LDM_coHighSpdP local single; V_LDM_coCSTI local single; V_LDM_coCSTP local; V_LDM_stBrkArbMode_en output; K_LDM_coDecelParalCtrlCST_I parameter; K_LDM_coDecelParalCtrlCST_P parameter; V_LDM_coEbrSlfBrkP local; V_LDM_coEbrSlfBrkI local; K_LDM_coDecelParalCtrlEbrSB_I parameter; K_LDM_coDecelParalCtrlEbrSB_P parameter; V_LDM_coLowSpdI local; V_LDM_coLowSpdP local; K_LDM_coDecelParalCtrlHighSpd_I parameter; K_LDM_coDecelParalCtrlLowSpd_I parameter; K_LDM_coDecelParalCtrlHighSpd_P parameter; K_LDM_coDecelParalCtrlLowSpd_P parameter; K_LDM_coDecelCtrlCl2OlLim parameter; K_LDM_coDecelCtrlHigh2LowLim parameter; K_LDM_coDecelCtrlLow2HighLim parameter; K_LDM_coDecelCtrlOl2ClLim parameter; K_LDM_blClsLoopCtrlEnable_bl parameter; V_LDM_stClsLoopEnable local; V_LDM_aVehAccErr local; V_LDM_aVehAccDecLong output single; V_LDM_stBrkSrcMode_en output

== stateflow chart LDM_Controller/Parallel-Hybird Controller/VehOritArb ==
  state Normal
    state Park
      V_LDM_stVehFwBw_en = LDMVehFwBw_en_t.Park;
    state Backward
      V_LDM_stVehFwBw_en = LDMVehFwBw_en_t.Backward;
    state Null
      V_LDM_stVehFwBw_en = LDMVehFwBw_en_t.Null;
    state Forward
      V_LDM_stVehFwBw_en = LDMVehFwBw_en_t.Forward;
    (default) -> (junction 33)
    (junction 33) -> Park [order 1] : [V_DBR_stTrShftLvrPos_en == TrShftLvrPos_en_t.ParkRange]
    Park -> Normal : [V_DBR_stTrShftLvrPos_en ~= TrShftLvrPos_en_t.ParkRange]
    (junction 33) -> (junction 44) [order 2]
    (junction 44) -> Backward [order 1] : [V_DBR_stTrShftLvrPos_en == TrShftLvrPos_en_t.ReverseRange]
    Backward -> Normal : [V_DBR_stTrShftLvrPos_en ~= TrShftLvrPos_en_t.ReverseRange]
    (junction 44) -> (junction 48) [order 2]
    (junction 48) -> Null [order 1] : [V_DBR_stTrShftLvrPos_en == TrShftLvrPos_en_t.BetweenRange || ...
        | V_DBR_stTrShftLvrPos_en == TrShftLvrPos_en_t.NeutralRange || ...
        | V_DBR_stTrShftLvrPos_en == TrShftLvrPos_en_t.Unknown]
    Null -> Normal : [V_DBR_stTrShftLvrPos_en ~= TrShftLvrPos_en_t.BetweenRange && ...
        | V_DBR_stTrShftLvrPos_en ~= TrShftLvrPos_en_t.NeutralRange && ...
        | V_DBR_stTrShftLvrPos_en ~= TrShftLvrPos_en_t.Unknown]
    (junction 48) -> (junction 41) [order 2]
    Forward -> Normal : [V_DBR_stTrShftLvrPos_en <4 || V_DBR_stTrShftLvrPos_en >11]
    (junction 41) -> Forward : % V_DBR_stTrShftLvrPos_en >=4 && V_DBR_stTrShftLvrPos_en<=11
  state Error
    V_LDM_stVehFwBw_en = LDMVehFwBw_en_t.Error;
  (default) -> (junction 35)
  (junction 35) -> Normal [order 1] : [V_DBR_vldTrShftLvrPosVD_bl == false]
  (junction 35) -> Error [order 2] : % V_DBR_vldTrShftLvrPosVD_bl == true
  Error -> Normal : [V_DBR_vldTrShftLvrPosVD_bl == false]
  Normal -> Error : [V_DBR_vldTrShftLvrPosVD_bl == true]
  data: V_DBR_vldTrShftLvrPosVD_bl input boolean; V_DBR_stTrShftLvrPos_en input Enum: TrShftLvrPos_en_t; V_LDM_stVehFwBw_en output Enum: LDMVehFwBw_en_t
